simulink model "nonlinear_model"  (R2020b)
settings: Solver=VariableStepAuto  StartTime=0.0  StopTime=10.0  RelTol=1e-3
undefined symbols (not defined in the file): C_l
settings Model: Creator=mahdi  LastModifiedBy=mahdi
settings DebuggingCC: SFMachineParentedDataDiag=error

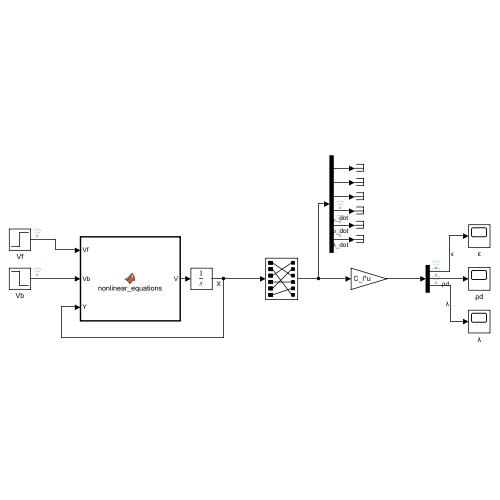
[thumbnail: Simulink's stored preview of the top-level diagram]
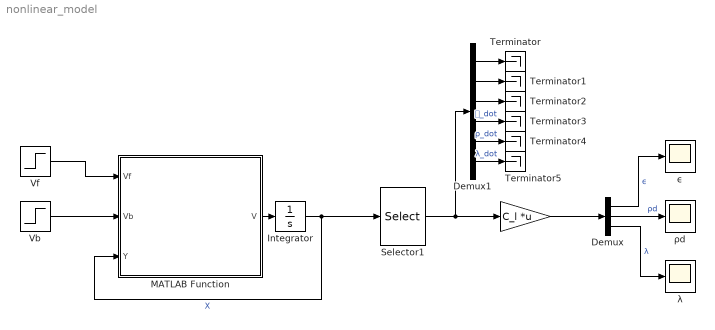
== system nonlinear_model ==
  " " : Gain  Gain=C_l  Multiplication=Matrix(K*u)
  Demux : Demux  Outputs=3
  Demux1 : Demux  Outputs=6
  Integrator : Integrator
  MATLAB Function : MATLAB Function  TreatAsAtomicUnit=on
  Selector1 : Selector  InputPortWidth=6  IndexOptions=Index vector (dialog)  Indices=[3,5,1,4,6,2]  OutputSizes=1
  Terminator{,1..5} (6 alike) : Terminator
  Vb : Step  After=-10  SampleTime=0
  Vf : Step  After=10  SampleTime=0
  λ : Scope
  ρd : Scope
  ϵ : Scope
  wires:
  Vf/1 -> MATLAB Function/1(Vf)
  Vb/1 -> MATLAB Function/2(Vb)
  Demux/1 -> ϵ/1  "ϵ"
  Demux1/6 -> Terminator5/1  "λ_dot"
  Demux/3 -> λ/1  "λ"
  Demux1/1 -> Terminator/1
  Demux1/5 -> Terminator4/1  "ρ_dot"
  Demux/2 -> ρd/1  "ρd"
  " "/1 -> Demux/1
  Demux1/2 -> Terminator1/1
  Demux1/4 -> Terminator3/1  "𝜖_dot"
  Demux1/3 -> Terminator2/1
  Integrator/1 -> Selector1/1, MATLAB Function/3(Y)  "X"
  MATLAB Function/1(V) -> Integrator/1
  Selector1/1 -> Demux1/1, " "/1

== matlab function nonlinear_model/MATLAB Function ==
  data: Vf input size=1; Vb input size=1; Y input size=6; V output size=6
function V = nonlinear_equations(Vf,Vb,Y)
%NONLINEAR_EQUATIONS
%    V = NONLINEAR_EQUATIONS(Vf,Vb,Y)

%    This function was generated by the Symbolic Math Toolbox version 9.0.
%    25-Jan-2022 22:45:14

t2 = Y(2);
t3 = Y(3);
t4 = Y(4);
t5 = Y(5);
t6 = Y(6);
t7 = cos(t3);
t8 = cos(t5);
t9 = sin(t3);
t10 = sin(t5);
t11 = t2.^2;
t12 = t7.^2;
t13 = t8.^2;
t14 = t8.^3;
t15 = 1.0./t12;
mt1 = [t2,t15.*(Vb.*t9.*-1.296935125776e+12+Vb.*t10.*4.80886057872e+12+Vf.*t9.*1.296935125776e+12-Vf.*t10.*4.80886057872e+12+Vb.*t9.*t13.*5.4285432876e+10-Vb.*t10.*t13.*2.0128306572e+11-Vf.*t9.*t13.*5.4285432876e+10+Vf.*t10.*t13.*2.0128306572e+11+t7.*t8.*t10.*1.567923921279e+12-t8.*t10.*t12.*1.567923921279e+12+Vb.*t7.*t8.*t10.*2.0128306572e+11+Vf.*t7.*t8.*t10.*2.0128306572e+11-t2.*t4.*t7.*t9.*1.26863517017056e+14+t4.*t6.*t7.*t13.*5.310088994098e+12+t2.*t4.*t7.*t9.*t13.*5.310088994098e+12-t2.*t6.*t8.*t10.*t12.*5.310088994098e+12-t8.*t9.*t10.*t11.*t12.*5.310088994098e+12).*-1.576497362698274e-14,t4];
mt2 = [((t7.*3.5891399884728e+13-t12.*3.5891399884728e+13+Vb.*t7.*4.607577513e+12+Vb.*t8.*2.0128306572e+11-Vb.*t14.*2.0128306572e+11+Vf.*t7.*4.607577513e+12-Vf.*t8.*2.0128306572e+11+Vf.*t14.*2.0128306572e+11+t7.*t13.*1.567923921279e+12-t12.*t13.*1.567923921279e+12+Vb.*t7.*t13.*2.0128306572e+11+Vf.*t7.*t13.*2.0128306572e+11+t2.*t6.*t12.*5.310088994098e+12-t9.*t11.*t12.*5.8121669514424e+13-Vb.*t8.*t9.*t10.*5.4285432876e+10+Vf.*t8.*t9.*t10.*5.4285432876e+10-t2.*t6.*t12.*t13.*5.310088994098e+12-t9.*t11.*t12.*t13.*5.310088994098e+12-t4.*t6.*t7.*t8.*t10.*5.310088994098e+12-t2.*t4.*t7.*t8.*t9.*t10.*5.310088994098e+12).*1.576497362698274e-14)./t7,t6];
mt3 = [t15.*(Vb.*-8.229961227637555e+16+Vf.*8.229961227637555e+16-Vb.*t12.*1.801623615426789e+18+Vb.*t13.*3.44479071401216e+15+Vf.*t12.*1.801623615426789e+18-Vf.*t13.*3.44479071401216e+15+Vb.*t9.*t10.*3.051558657438515e+17-Vb.*t12.*t13.*3.44479071401216e+15-Vf.*t9.*t10.*3.051558657438515e+17+Vf.*t12.*t13.*3.44479071401216e+15-t2.*t4.*t7.*8.050378199351165e+18-Vb.*t9.*t10.*t13.*1.277281950139392e+16+Vf.*t9.*t10.*t13.*1.277281950139392e+16+t2.*t4.*t7.*t13.*3.369623172984996e+17+t7.*t8.*t9.*t10.*9.949574827260314e+16-t8.*t9.*t10.*t12.*9.949574827260314e+16-t8.*t10.*t11.*t12.*3.369623172984996e+17+t2.*t4.*t7.^3.*t13.*7.713415882051944e+18+t4.^2.*t8.*t10.*t12.*4.025189099675582e+18-t8.*t10.*t11.*1.0./t15.^2.*3.688226782376886e+18+Vb.*t7.*t8.*t9.*t10.*1.277281950139392e+16+Vf.*t7.*t8.*t9.*t10.*1.277281950139392e+16+t4.*t6.*t7.*t9.*t13.*3.369623172984996e+17-t2.*t6.*t8.*t9.*t10.*t12.*3.369623172984996e+17).*2.484355331481322e-19];
V = reshape([mt1,mt2,mt3],6,1);
